simulink model "untitled"  (R2018b)
settings: Solver=VariableStepAuto  StartTime=0.0  StopTime=100  RelTol=1e-3
settings Model: Creator=ali  LastModifiedBy=ali

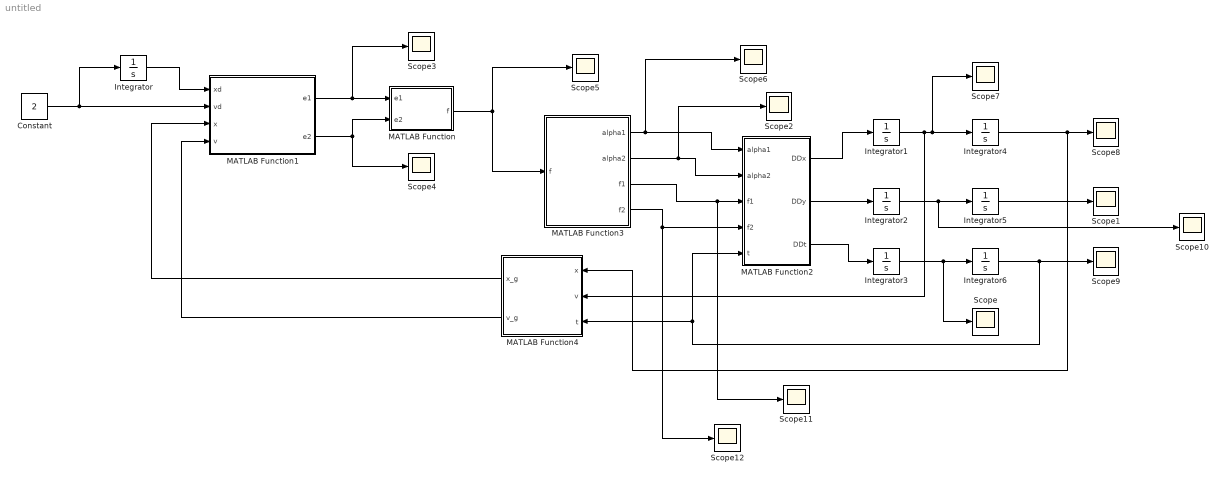
== system untitled ==
  Constant : Constant  Value=2
  Integrator{,1..4,6} (6 alike) : Integrator
  Integrator5 : Integrator  InitialCondition=10
  MATLAB Function : MATLAB Function  TreatAsAtomicUnit=on
  MATLAB Function1 : MATLAB Function  TreatAsAtomicUnit=on
  MATLAB Function2 : MATLAB Function  TreatAsAtomicUnit=on
  MATLAB Function3 : MATLAB Function  TreatAsAtomicUnit=on
  MATLAB Function4 : MATLAB Function  TreatAsAtomicUnit=on
  Scope{,1..12} (13 alike) : Scope
  wires:
  MATLAB Function1/1(e1) -> Scope3/1, MATLAB Function/1(e1)
  MATLAB Function1/2(e2) -> Scope4/1, MATLAB Function/2(e2)
  Constant/1 -> Integrator/1, MATLAB Function1/2(vd)
  Integrator/1 -> MATLAB Function1/1(xd)
  MATLAB Function2/1(DDx) -> Integrator1/1
  MATLAB Function2/2(DDy) -> Integrator2/1
  MATLAB Function/1(f) -> Scope5/1, MATLAB Function3/1(f)
  MATLAB Function3/1(alpha1) -> Scope6/1, MATLAB Function2/1(alpha1)
  MATLAB Function2/3(DDt) -> Integrator3/1
  Integrator1/1 -> MATLAB Function4/2(v), Scope7/1, Integrator4/1
  Integrator2/1 -> Scope10/1, Integrator5/1
  Integrator3/1 -> Scope/1, Integrator6/1
  Integrator6/1 -> MATLAB Function4/3(t), MATLAB Function2/5(t), Scope9/1
  Integrator5/1 -> Scope1/1
  Integrator4/1 -> MATLAB Function4/1(x), Scope8/1
  MATLAB Function4/1(x_g) -> MATLAB Function1/3(x)
  MATLAB Function4/2(v_g) -> MATLAB Function1/4(v)
  MATLAB Function3/2(alpha2) -> Scope2/1, MATLAB Function2/2(alpha2)
  MATLAB Function3/3(f1) -> MATLAB Function2/3(f1), Scope11/1
  MATLAB Function3/4(f2) -> Scope12/1, MATLAB Function2/4(f2)

== matlab function untitled/MATLAB Function1 ==
  data: xd input; e1 output; vd input; x input; v input; e2 output
function [e1,e2] = fcn(xd,vd,x,v)

k1 = 1;

e1 = xd - x;
u = vd + k1*e1;
e2 = u - v;

end

== matlab function untitled/MATLAB Function ==
  data: e1 input; f output; e2 input
function f = fcn(e1,e2)

k1 = 1;
k2 = 1;

f = k2*e2 - (k1^2)*e1;

end

== matlab function untitled/MATLAB Function2 ==
  data: alpha1 input; alpha2 input; f1 input; f2 input; DDx output; DDy output; DDt output; t input
function [DDx,DDy,DDt] = fcn(alpha1,alpha2,f1,f2,t)

g= 9.81;
m = 1;
d = 1;
I = 0.1;

DDy = (1/m)*( f1*sin(alpha1+t) + f2*sin(alpha2+t) - (m*g));
DDx = (1/m)*( f1*cos(alpha1+t) + f2*cos(alpha2+t) );
DDt = (d/I)*( f1*sin(alpha1) - f2*sin(alpha2) );

end

== matlab function untitled/MATLAB Function3 ==
  data: f input; alpha1 output; alpha2 output; f1 output; f2 output
function [alpha1,alpha2,f1,f2] = fcn(f)

g = 9.81;
m=1;
S = f/g;
alpha = abs(atan(1/S));
P = abs(m*g/sin(alpha));

alpha1 = alpha;
alpha2 = alpha;
f1 = P/2;
f2 = P/2;

end

== matlab function untitled/MATLAB Function4 ==
  data: x input; x_g output; v_g output; v input; t input
function [x_g,v_g] = fcn(x,v,t)

x_g = x / cos(t);
v_g = v / cos(t);

end
